simulink model "MultiRigidBody"  (R2019a)
settings: Solver=ode3  StartTime=0.0  StopTime=Time  FixedStep=Ts  RelTol=1e-3
values from neighbouring files (symbols this model uses):
  a1 = 0.2634    [start.m]
  a2 = 1.6279    [start.m]
  a3 = 25.6488    [start.m]
  b1 = 0.531    [start.m]
  b2 = 5.3292    [start.m]
  b3 = 0.531    [start.m]
  b4 = 0.1157    [start.m]
  ce = 0.10    (= 0.1)    [start.m]
  ce1 = 0.053    [start.m]
  cp = 0.4804    [start.m]
  cp1 = 0.274    [start.m]
  ct = 0.3410    (= 0.341)    [start.m]
  ct1 = 0.048    [start.m]
  dot_q0 = [0 0 0]'    [start.m]
  g = 9.81    [start.m]
  I_e = 1.469    [start.m]
  I_t = 0.0319    [start.m]
  lcd = 0.10    (= 0.1)    [start.m]
  ldf = 0.17    [start.m]
  loc = 0.78    [start.m]
  m = (-mc*lob + mh *loc + mb*loa)/loc    (= 0.547587958974)    [start.m]
  mh = 1.8    [start.m]
  q0 = [0 0 0]'    [start.m]
  Ts = 0.005    [caldot_for_17.m]    (also in start.m)
libraries: dspsrcs4 x4
settings Model: Creator=chen  LastModifiedBy=DELL
settings DataIOCC: ReturnWorkspaceOutputs=off
settings DebuggingCC: PregeneratedLibrarySubsystemCodeDiagnostic=none  ArithmeticOperatorsInVariantConditions=warning
settings SFSimCC: SimUseLocalCustomCode=off
settings RTWCC: RTWUseLocalCustomCode=off

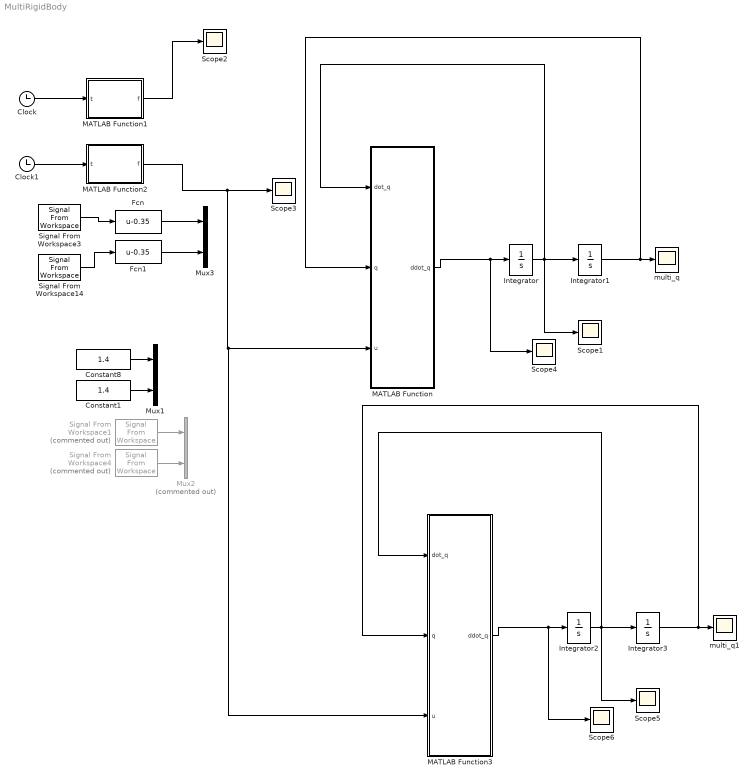
== system MultiRigidBody ==
  Clock : Clock
  Clock1 : Clock
  Constant1 : Constant  Value=1.4
  Constant8 : Constant  Value=1.4
  Fcn : Fcn  Expr=u-0.35
  Fcn1 : Fcn  Expr=u-0.35
  Integrator : Integrator  InitialCondition=dot_q0
  Integrator1 : Integrator  InitialCondition=q0
  Integrator2 : Integrator  InitialCondition=dot_q0
  Integrator3 : Integrator  InitialCondition=q0
  MATLAB Function : MATLAB Function  TreatAsAtomicUnit=on
  MATLAB Function1 : MATLAB Function  TreatAsAtomicUnit=on
  MATLAB Function2 : MATLAB Function  TreatAsAtomicUnit=on
  MATLAB Function3 : MATLAB Function  TreatAsAtomicUnit=on
  Mux1 : Mux  Inputs=2
  Mux2 : Mux  Commented=on  Inputs=2
  Mux3 : Mux  Inputs=2
  Scope{1..6} (6 alike) : Scope
  Signal From Workspace1 : dspsrcs4/Signal From Workspace  Commented=on  X=f1  Ts=Ts  nsamps=1  OutputAfterFinalValue=Setting to zero  ignoreOrWarnInputAndFrameLengths=off  OutputFrames=on
  Signal From Workspace14 : dspsrcs4/Signal From Workspace  X=F1  Ts=Ts  nsamps=1  OutputAfterFinalValue=Setting to zero  ignoreOrWarnInputAndFrameLengths=off  OutputFrames=on
  Signal From Workspace3 : dspsrcs4/Signal From Workspace  X=F2  Ts=Ts  nsamps=1  OutputAfterFinalValue=Setting to zero  ignoreOrWarnInputAndFrameLengths=off  OutputFrames=on
  Signal From Workspace4 : dspsrcs4/Signal From Workspace  Commented=on  X=f2  Ts=Ts  nsamps=1  OutputAfterFinalValue=Setting to zero  ignoreOrWarnInputAndFrameLengths=off  OutputFrames=on
  multi_q : Scope
  multi_q1 : Scope
  wires:
  MATLAB Function/1(ddot_q) -> Scope4/1, Integrator/1
  Integrator/1 -> MATLAB Function/1(dot_q), Scope1/1, Integrator1/1
  Integrator1/1 -> MATLAB Function/2(q), multi_q/1
  Signal From Workspace14/1 -> Fcn1/1
  Signal From Workspace3/1 -> Fcn/1
  Clock/1 -> MATLAB Function1/1(t)
  Clock1/1 -> MATLAB Function2/1(t)
  Fcn/1 -> Mux3/1
  Fcn1/1 -> Mux3/2
  Constant8/1 -> Mux1/1
  Constant1/1 -> Mux1/2
  Signal From Workspace1/1 -> Mux2/1
  Signal From Workspace4/1 -> Mux2/2
  MATLAB Function1/1(f) -> Scope2/1
  MATLAB Function2/1(f) -> MATLAB Function3/3(u), MATLAB Function/3(u), Scope3/1
  Integrator2/1 -> MATLAB Function3/1(dot_q), Scope5/1, Integrator3/1
  MATLAB Function3/1(ddot_q) -> Scope6/1, Integrator2/1
  Integrator3/1 -> MATLAB Function3/2(q), multi_q1/1

== matlab function MultiRigidBody/MATLAB Function1 ==
  data: t input; f output
function f = fcn(t)
f1 = 0;
f2 = 0;
if t>=0&&t<30
    f1 = 1.5;
    f2 = 1.5;
elseif t>=30
    f1 = 1.7;
    f2 = 1.2;
end
f = [f1;f2];

== matlab function MultiRigidBody/MATLAB Function ==
  data: dot_q input; q input; u input; ddot_q output; ce parameter; I_t parameter; I_e parameter; loc parameter; lcd parameter; ldf parameter; mh parameter; m parameter; g parameter; a1 parameter; a2 parameter; b1 parameter; a3 parameter; b2 parameter; ct parameter; b3 parameter; b4 parameter; cp parameter; cp1 parameter; ce1 parameter; ct1 parameter
function ddot_q = fcn(dot_q,q,u,ce, I_t, I_e, loc, lcd, ldf, mh, m, g, a1, a2, b1, a3, b2, ct, b3, b4, cp, cp1, ce1, ct1)
I_psi = I_e;
%psai = q(1);
epsilon = q(2);
theta = q(3);
dot_psai = dot_q(1);
dot_epsilon = dot_q(2);
dot_theta = dot_q(3);

fs = u(1) + u(2); 
fd = u(1) - u(2);

%未辨识
% ddot_q1 = (loc*cos(epsilon)*sin(theta)*fs - ldf * sin(theta)*sin(epsilon)*fd)/I_psi - cp1*dot_psai;
% ddot_q2 = (-mh * g*lcd*cos(theta)*sin(epsilon) - m*g*loc*cos(epsilon) + loc * cos(theta)*fs)/I_e - ce1*dot_epsilon;
% ddot_q3 = ( -mh *g* lcd *cos(epsilon)*sin(theta) + ldf*fd)/I_t - ct1*dot_theta;

%辨识方程
ddot_q1 = b3*cos(epsilon)*sin(theta)*fs - b4 * sin(theta)*sin(epsilon)*fd - cp*dot_psai;
ddot_q2 = -a1*cos(theta)*sin(epsilon) - a2*cos(epsilon) + b1 * cos(theta)*fs - ce*dot_epsilon;
ddot_q3 = -a3*cos(epsilon)*sin(theta) + b2*fd - ct*dot_theta;

% % % ddot_q1 = -b3*cos(epsilon)*sin(theta)*fs + b4 * cos(theta)*sin(epsilon)*fd ;
% % % ddot_q2 = -a1*cos(theta)*sin(epsilon) + a2*cos(epsilon) - b1 * cos(theta)*fs ;
% % % ddot_q3 = -a3*cos(epsilon)*sin(theta) + b2*fd ;
ddot_q = [ddot_q1;ddot_q2;ddot_q3];

== matlab function MultiRigidBody/MATLAB Function2 ==
  data: t input; f output
function f = fcn(t)
f1 = 0;
f2 = 0;
if t>0&&t<25
    f1 = 1.7;
    f2 = 1.2;
elseif t>=25
    f1 = 1.3;
    f2 = 1.6;
end
f = [f1;f2];

== matlab function MultiRigidBody/MATLAB Function3 ==
  data: dot_q input; q input; u input; ddot_q output; ce parameter; I_t parameter; I_e parameter; loc parameter; lcd parameter; ldf parameter; mh parameter; m parameter; g parameter; a1 parameter; a2 parameter; b1 parameter; a3 parameter; b2 parameter; ct parameter; b3 parameter; b4 parameter; cp parameter; cp1 parameter; ce1 parameter; ct1 parameter
function ddot_q = fcn(dot_q,q,u,ce, I_t, I_e, loc, lcd, ldf, mh, m, g, a1, a2, b1, a3, b2, ct, b3, b4, cp, cp1, ce1, ct1)
I_psi = I_e;
%psai = q(1);
epsilon = q(2);
theta = q(3);
dot_psai = dot_q(1);
dot_epsilon = dot_q(2);
dot_theta = dot_q(3);

fs = u(1) + u(2); 
fd = u(1) - u(2);

%未辨识
ddot_q1 = (loc*cos(epsilon)*sin(theta)*fs - ldf * sin(theta)*sin(epsilon)*fd)/I_psi - cp1*dot_psai;
ddot_q2 = (-mh * g*lcd*cos(theta)*sin(epsilon) - m*g*loc*cos(epsilon) + loc * cos(theta)*fs)/I_e - ce1*dot_epsilon;
ddot_q3 = ( -mh *g* lcd *cos(epsilon)*sin(theta) + ldf*fd)/I_t - ct1*dot_theta;

%辨识方程
% ddot_q1 = b3*cos(epsilon)*sin(theta)*fs - b4 * sin(theta)*sin(epsilon)*fd - cp*dot_psai;
% ddot_q2 = -a1*cos(theta)*sin(epsilon) - a2*cos(epsilon) + b1 * cos(theta)*fs - ce*dot_epsilon;
% ddot_q3 = -a3*cos(epsilon)*sin(theta) + b2*fd - ct*dot_theta;

% % % ddot_q1 = -b3*cos(epsilon)*sin(theta)*fs + b4 * cos(theta)*sin(epsilon)*fd ;
% % % ddot_q2 = -a1*cos(theta)*sin(epsilon) + a2*cos(epsilon) - b1 * cos(theta)*fs ;
% % % ddot_q3 = -a3*cos(epsilon)*sin(theta) + b2*fd ;
ddot_q = [ddot_q1;ddot_q2;ddot_q3];
